simulink model "reClarke"  (R2022b)
settings: Solver=VariableStepAuto  StartTime=0.0  StopTime=10.0  RelTol=1e-3
settings Model: Creator=15403  LastModifiedBy=15403

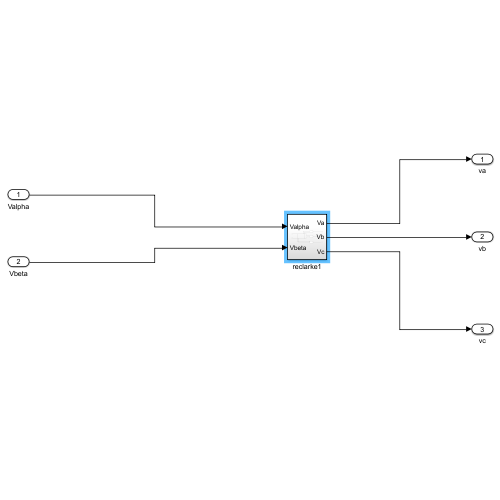
[thumbnail: Simulink's stored preview of the top-level diagram]
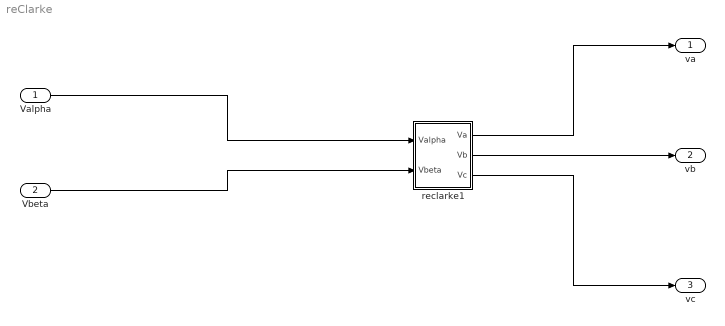
== system reClarke ==
  Valpha : Inport
  Vbeta : Inport  Port=2
  reclarke1 : Subsystem
  va : Outport
  vb : Outport  Port=2
  vc : Outport  Port=3
  wires:
  Valpha/1 -> reclarke1/1(Valpha)
  Vbeta/1 -> reclarke1/2(Vbeta)
  reclarke1/1(Va) -> va/1
  reclarke1/2(Vb) -> vb/1
  reclarke1/3(Vc) -> vc/1

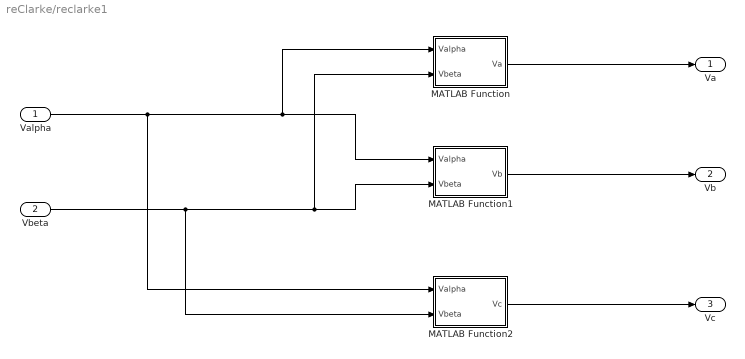
== system reClarke/reclarke1 ==
  Valpha : Inport
  Vbeta : Inport  Port=2
  MATLAB Function : MATLAB Function  TreatAsAtomicUnit=on
  MATLAB Function1 : MATLAB Function  TreatAsAtomicUnit=on
  MATLAB Function2 : MATLAB Function  TreatAsAtomicUnit=on
  Va : Outport
  Vb : Outport  Port=2
  Vc : Outport  Port=3
  wires:
  Valpha/1 -> MATLAB Function2/1(Valpha), MATLAB Function/1(Valpha), MATLAB Function1/1(Valpha)
  MATLAB Function1/1(Vb) -> Vb/1
  Vbeta/1 -> MATLAB Function2/2(Vbeta), MATLAB Function/2(Vbeta), MATLAB Function1/2(Vbeta)
  MATLAB Function/1(Va) -> Va/1
  MATLAB Function2/1(Vc) -> Vc/1

== matlab function reClarke/reclarke1/MATLAB Function1 ==
  data: Valpha input; Vb output; Vbeta input
function Vb = fcn(Valpha, Vbeta)

Vb = -Valpha * sind(30) + Vbeta * cosd(30);

== matlab function reClarke/reclarke1/MATLAB Function2 ==
  data: Valpha input; Vc output; Vbeta input
function Vc = fcn(Valpha, Vbeta)

Vc = -Valpha * sind(30) - Vbeta * cosd(30);

== matlab function reClarke/reclarke1/MATLAB Function ==
  data: Valpha input; Va output; Vbeta input
function Va = fcn(Valpha, Vbeta)

Va = Valpha;
